simulink model "ball_on_beam_observer_feedback_template"  (R2024a)
settings: Solver=VariableStepAuto  StartTime=0.0  StopTime=20  RelTol=1e-3
undefined symbols (not defined in the file or in its folder): A_num, b_u_num, K, Ll
libraries: vrlib x4
settings Model: Creator=muellerb  LastModifiedBy=boraderici
settings DebuggingCC: UnconnectedInputMsg=warning  UnconnectedOutputMsg=warning  UnconnectedLineMsg=warning
settings ModelReferenceCC: EnableRefExpFcnMdlSchedulingChecks=on
settings RTWCC: GPUComputeCapability=3.5  DLArmComputeVersion=19.05

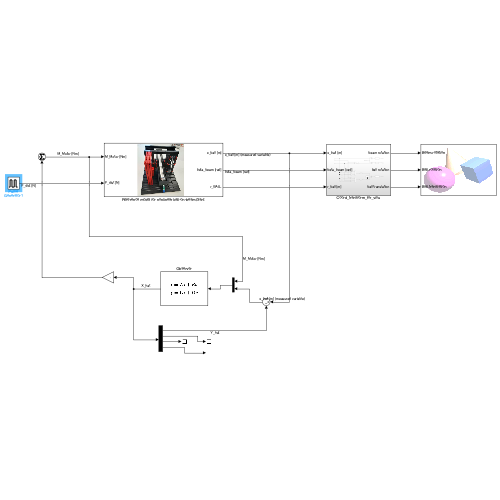
[thumbnail: Simulink's stored preview of the top-level diagram]
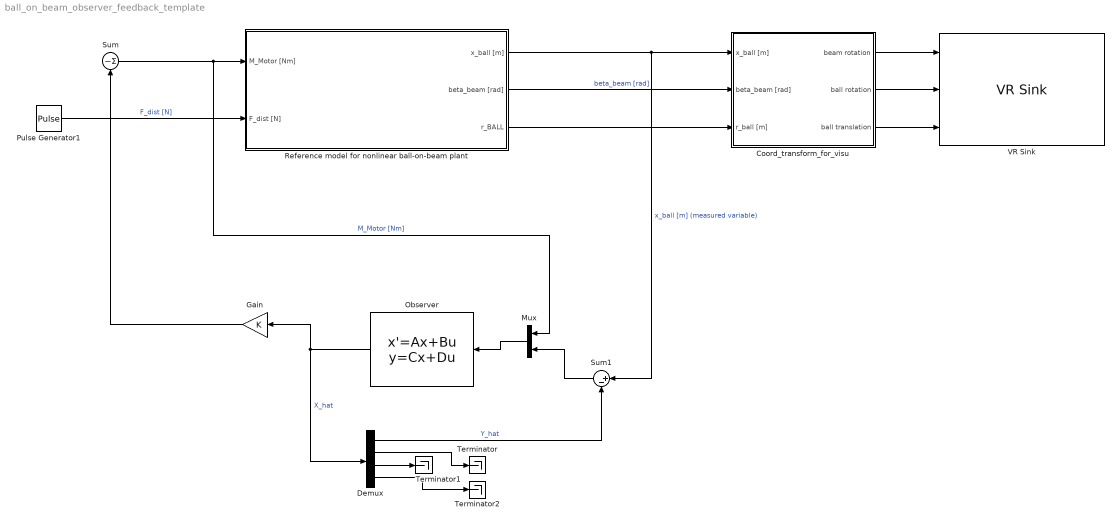
== system ball_on_beam_observer_feedback_template ==
  Coord_transform_for_visu : Subsystem
  Demux : Demux
  Gain : Gain  Gain=K
  Mux : Mux  Inputs=2
  Observer : StateSpace  A=A_num  B=[b_u_num Ll]  C=eye(4,4)  D=zeros(4,2)  InitialCondition=[0,0,0,0]
  Pulse Generator1 : DiscretePulseGenerator  PulseType=Time based  Amplitude=1.25  Period=12  PulseWidth=0.25  PhaseDelay=0.25
  Reference model for nonlinear ball-on-beam plant : Subsystem  mask(Nonlinear BALL_ON_BEAM model){r_BALL=0.0125, J_BALL=4.00e-06, m_BALL=0.064, G=9.81, J_BEAM=2.9e-3}
      mask prompts: r_BALL "Radius of the ball r_ball [m]"; J_BALL "Moment of inertia of the ball J_ball [kgm^2] (with respect to axis of symmetry)"; m_BALL "Mass of ball m_ball [kg]"; G "Gravity acceleration g [m/s^2]"; J_BEAM "Moment of inertia of the beam J_beam [kgm^2] (with respect to the axis of rotation)"
      mask help: Nonlinear model of ball-on-beam setup (without restrictions on input or state variables)
      mask Display: image('$imagefile'); % Use "Edit Image" on toolstrip to change.
  Sum : Sum  Inputs=|-
  Sum1 : Sum  Inputs=|+-
  Terminator : Terminator
  Terminator1 : Terminator
  Terminator2 : Terminator
  VR Sink : vrlib/VR Sink  InstantiateOnLoad=on  SampleTime=0.1  ViewEnable=on  RemoteChange=off  RemoteView=off  FieldsWritten=Beam.rotation.4.1.1.double#Ball.rotation.4.1.1.double#Ball.translation.3.1.1.double  WorldFileName=Ball_on_beam.wrl  AutoView=on  VideoDimensions=[]  AllowVariableSize=off  FigureProperties="{'Position', 'Name', 'Viewpoint', 'CameraBound', 'CameraDirection', 'CameraPosition', 'CameraUpVector', 'ZoomFactor', 'Antialiasing', 'Headlight', 'Lighting', 'Sound', 'StatusBar', 'Stereo3D', 'Stereo3DCameraOffset', 'Stereo3DHIT', 'ToolBar', 'Textures', 'Transparency', 'Triad', 'Wireframe', 'NavZones', 'NavMode', 'NavSpeed', 'CaptureFileFormat', 'CaptureFileName', 'Record2DCompressMethod', 'Record2DCompressQuality', 'Record2D', 'Record2DFileName', 'Record2DFPS', 'NavPanel'; [5.0000000000000000e+00   1.0300000000000000e+02   5.7600000000000000e+02   3.5000000000000000e+02], '', '_untitled_1', 'on', [3.8941834230865069e-01   0.0000000000000000e+00  -9.2106099400288599e-01], [-1.0778285057537843e+01   0.0000000000000000e+00  -1.6897252106831864e+01], [0.0000000000000000e+00   1.0000000000000000e+00   0.0000000000000000e+00], [1.0000000000000000e+00], 'on', 'on', 'on', 'on', 'on', 'off', [1.0000000149011612e-01], [0.0000000000000000e+00], 'on', 'on', 'on', 'none', 'off', 'off', 'fly', 'normal', 'tif', '%f_anim_%n.tif', 'auto', [7.5000000000000000e+01], 'off', '%f_anim_%n.avi', 'auto', 'halfbar'}"
  wires:
  Pulse Generator1/1 -> Reference model for nonlinear ball-on-beam plant/2(F_dist [N])  "F_dist [N]"
  Reference model for nonlinear ball-on-beam plant/3(r_BALL) -> Coord_transform_for_visu/3(r_ball [m])
  Reference model for nonlinear ball-on-beam plant/1(x_ball [m]) -> Sum1/1, Coord_transform_for_visu/1(x_ball [m])  "x_ball [m] (measured variable)"
  Reference model for nonlinear ball-on-beam plant/2(beta_beam [rad]) -> Coord_transform_for_visu/2(beta_beam [rad])  "beta_beam [rad]"
  Sum/1 -> Mux/1, Reference model for nonlinear ball-on-beam plant/1(M_Motor [Nm])  "M_Motor [Nm]"
  Coord_transform_for_visu/1(beam rotation) -> VR Sink/1
  Coord_transform_for_visu/2(ball rotation) -> VR Sink/2
  Coord_transform_for_visu/3(ball translation) -> VR Sink/3
  Gain/1 -> Sum/1
  Observer/1 -> Gain/1, Demux/1  "X_hat"
  Demux/2 -> Terminator/1
  Demux/3 -> Terminator1/1
  Demux/4 -> Terminator2/1
  Demux/1 -> Sum1/2  "Y_hat"
  Sum1/1 -> Mux/2
  Mux/1 -> Observer/1

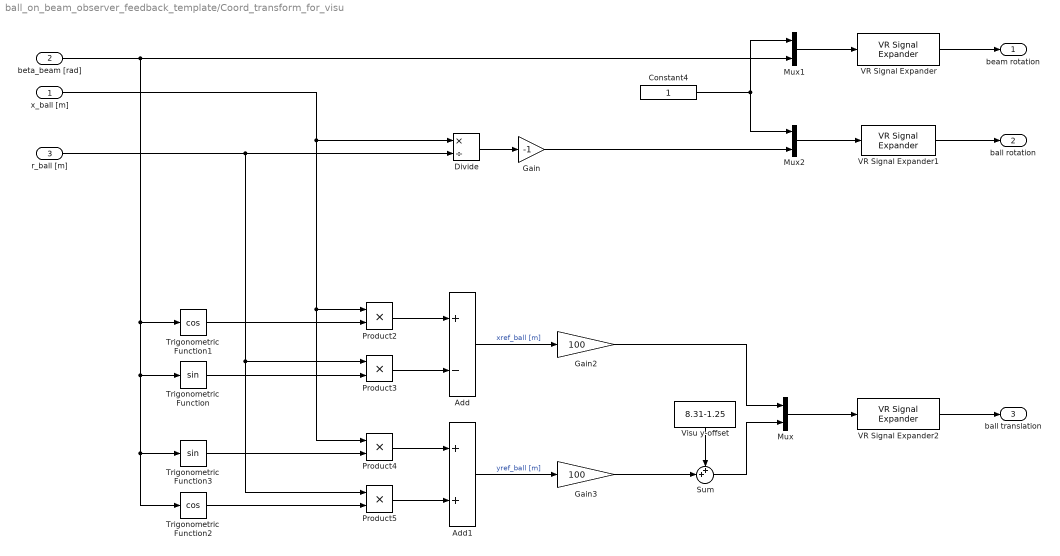
== system ball_on_beam_observer_feedback_template/Coord_transform_for_visu ==
  x_ball [m] : Inport
  beta_beam [rad] : Inport  Port=2
  r_ball [m] : Inport  Port=3
  Add : Sum  Inputs=+-
  Add1 : Sum
  Constant4 : Constant
  Divide : Product  Inputs=*/
  Gain : Gain  Gain=-1
  Gain2 : Gain  Gain=100
  Gain3 : Gain  Gain=100
  Mux : Mux  Inputs=2
  Mux1 : Mux  Inputs=2
  Mux2 : Mux  Inputs=2
  Product{2..5} (4 alike) : Product
  Sum : Sum  Inputs=++|
  Trigonometric Function : Trigonometry
  Trigonometric Function1 : Trigonometry  Operator=cos
  Trigonometric Function2 : Trigonometry  Operator=cos
  Trigonometric Function3 : Trigonometry
  VR Signal Expander : vrlib/VR Signal Expander  outwidth=4  outidx=[3 4]
  VR Signal Expander1 : vrlib/VR Signal Expander  outwidth=4  outidx=[3 4]
  VR Signal Expander2 : vrlib/VR Signal Expander  outwidth=3  outidx=[1 2]
  Visu y-offset : Constant  Value=8.31-1.25
  beam rotation : Outport
  ball rotation : Outport  Port=2
  ball translation : Outport  Port=3
  wires:
  r_ball [m]/1 -> Divide/2, Product5/1, Product3/1
  Add/1 -> Gain2/1  "xref_ball [m]"
  x_ball [m]/1 -> Product4/1, Product2/1, Divide/1
  beta_beam [rad]/1 -> Mux1/2, Trigonometric Function1/1, Trigonometric Function2/1, Trigonometric Function3/1, Trigonometric Function/1
  Mux/1 -> VR Signal Expander2/1
  VR Signal Expander/1 -> beam rotation/1
  VR Signal Expander2/1 -> ball translation/1
  Trigonometric Function3/1 -> Product4/2
  Add1/1 -> Gain3/1  "yref_ball [m]"
  Gain/1 -> Mux2/2
  Mux2/1 -> VR Signal Expander1/1
  Constant4/1 -> Mux2/1, Mux1/1
  Trigonometric Function2/1 -> Product5/2
  Mux1/1 -> VR Signal Expander/1
  Divide/1 -> Gain/1
  Product4/1 -> Add1/1
  Visu y-offset/1 -> Sum/1
  Product5/1 -> Add1/2
  Gain2/1 -> Mux/1
  Product3/1 -> Add/2
  Trigonometric Function1/1 -> Product2/2
  Trigonometric Function/1 -> Product3/2
  Sum/1 -> Mux/2
  VR Signal Expander1/1 -> ball rotation/1
  Gain3/1 -> Sum/2
  Product2/1 -> Add/1

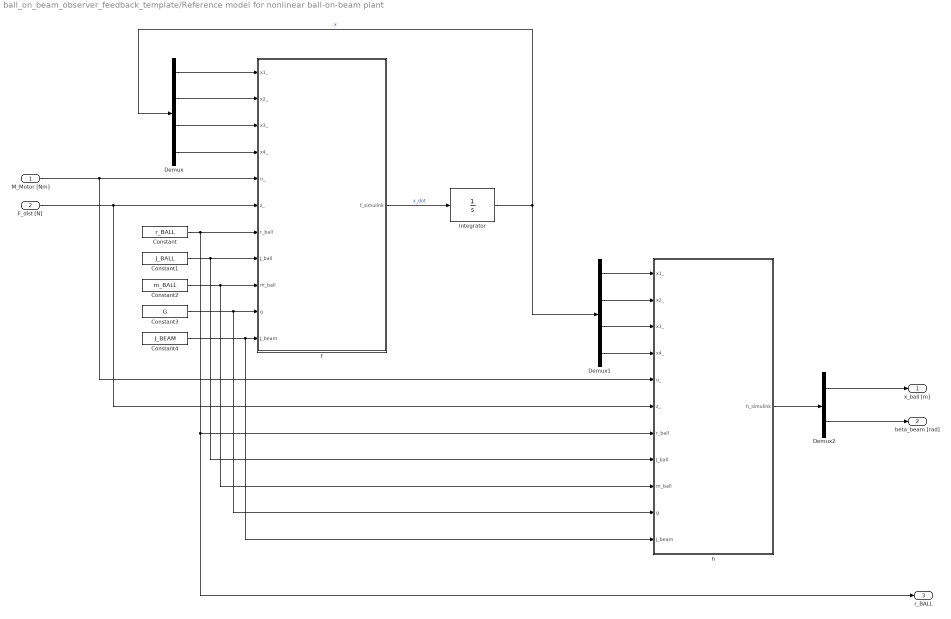
== system ball_on_beam_observer_feedback_template/Reference model for nonlinear ball-on-beam plant ==
  M_Motor [Nm] : Inport
  F_dist [N] : Inport  Port=2
  Constant : Constant  Value=r_BALL
  Constant1 : Constant  Value=J_BALL
  Constant2 : Constant  Value=m_BALL
  Constant3 : Constant  Value=G
  Constant4 : Constant  Value=J_BEAM
  Demux : Demux
  Demux1 : Demux
  Demux2 : Demux  Outputs=2
  Integrator : Integrator
  f : MATLAB Function  TreatAsAtomicUnit=on
  h : MATLAB Function  TreatAsAtomicUnit=on
  x_ball [m] : Outport
  beta_beam [rad] : Outport  Port=2
  r_BALL : Outport  Port=3
  wires:
  Demux2/1 -> x_ball [m]/1
  M_Motor [Nm]/1 -> h/5(u_), f/5(u_)
  f/1(f_simulink) -> Integrator/1  "x_dot"
  h/1(h_simulink) -> Demux2/1
  Demux/3 -> f/3(x3_)
  Constant1/1 -> h/8(J_ball), f/8(J_ball)
  Demux/1 -> f/1(x1_)
  Integrator/1 -> Demux/1, Demux1/1  "x"
  F_dist [N]/1 -> h/6(z_), f/6(z_)
  Demux1/1 -> h/1(x1_)
  Constant4/1 -> h/11(J_beam), f/11(J_beam)
  Constant3/1 -> h/10(g), f/10(g)
  Constant/1 -> r_BALL/1, h/7(r_ball), f/7(r_ball)
  Demux2/2 -> beta_beam [rad]/1
  Constant2/1 -> h/9(m_ball), f/9(m_ball)
  Demux/2 -> f/2(x2_)
  Demux/4 -> f/4(x4_)
  Demux1/2 -> h/2(x2_)
  Demux1/3 -> h/3(x3_)
  Demux1/4 -> h/4(x4_)

== matlab function ball_on_beam_observer_feedback_template/Reference model for nonlinear ball-on-beam plant/h ==
  data: x1_ input; h_simulink output; x2_ input; x3_ input; x4_ input; u_ input; z_ input; r_ball input; J_ball input; m_ball input; g input; J_beam input
function h_simulink = h(x1_,x2_,x3_,x4_,u_,z_,r_ball,J_ball,m_ball,g,J_beam)
%#codegen

%    This function was generated by the Symbolic Math Toolbox version 8.7.
%    28-Nov-2023 16:51:32

h_simulink = [x1_;...
    x3_];

== matlab function ball_on_beam_observer_feedback_template/Reference model for nonlinear ball-on-beam plant/f ==
  data: x1_ input; f_simulink output; x2_ input; x3_ input; x4_ input; u_ input; z_ input; r_ball input; J_ball input; m_ball input; g input; J_beam input
function f_simulink = f(x1_,x2_,x3_,x4_,u_,z_,r_ball,J_ball,m_ball,g,J_beam)
%#codegen

%    This function was generated by the Symbolic Math Toolbox version 8.7.
%    28-Nov-2023 16:51:32

t2 = cos(x3_);
t3 = sin(x3_);
t4 = m_ball.^2;
t5 = r_ball.^2;
t6 = x1_.^2;
t7 = x4_.^2;
t8 = m_ball.*t6;
t9 = J_beam+t8;
t10 = 1.0./t9;
f_simulink = [x2_;...
    (r_ball.*t10.*(J_ball.*u_+J_beam.*r_ball.*z_+m_ball.*t5.*u_+r_ball.*t8.*z_+r_ball.*t4.*t7.*x1_.^3+r_ball.^3.*t4.*t7.*x1_-J_beam.*g.*m_ball.*r_ball.*t3-J_ball.*g.*m_ball.*t2.*x1_+J_beam.*m_ball.*r_ball.*t7.*x1_+J_ball.*m_ball.*r_ball.*t7.*x1_-J_ball.*m_ball.*x1_.*x2_.*x4_.*2.0-g.*r_ball.*t3.*t4.*t6-g.*t2.*t4.*t5.*x1_-t4.*t5.*x1_.*x2_.*x4_.*2.0))./(J_ball+m_ball.*t5);x4_;t10.*(u_-g.*m_ball.*t2.*x1_+m_ball.*r_ball.*t7.*x1_-m_ball.*x1_.*x2_.*x4_.*2.0)];
